simulink model "lab10"  (R2022b)
settings: Solver=VariableStepAuto  StartTime=0.0  StopTime=50  RelTol=1e-3
settings Model: Creator=micha  LastModifiedBy=mateu

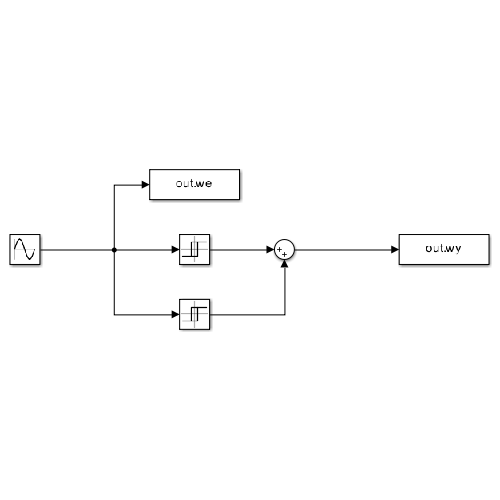
[thumbnail: Simulink's stored preview of the top-level diagram]
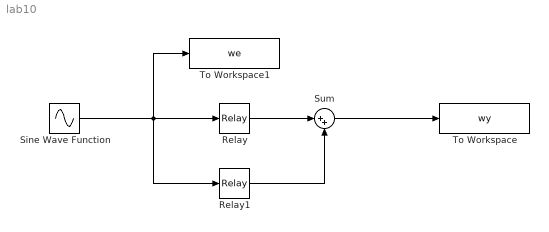
== system lab10 ==
  Relay : Relay  OnSwitchValue=0.073  OffSwitchValue=0.05  OnOutputValue=3
  Relay1 : Relay  OnSwitchValue=-0.05  OffSwitchValue=-0.073  OnOutputValue=0  OffOutputValue=-3
  Sine Wave Function : Sin  Amplitude=6  SampleTime=0
  Sum : Sum  Inputs=|++
  To Workspace : ToWorkspace  VariableName=wy  SampleTime=-1
  To Workspace1 : ToWorkspace  VariableName=we  SampleTime=-1
  wires:
  Sine Wave Function/1 -> To Workspace1/1, Relay1/1, Relay/1
  Relay1/1 -> Sum/2
  Relay/1 -> Sum/1
  Sum/1 -> To Workspace/1
